simulink model "rpi_dc_motor_control"  (R2014a)
settings: Solver=FixedStepDiscrete  StartTime=0.0  StopTime=5000  FixedStep=0.001  RelTol=1e-3
undefined symbols (not defined in the file): DiscIntNeverNeededParam
settings Model: SimulationMode=external  ExtModeTrigDuration=200000  Creator=krecmich  LastModifiedBy=ses
settings OptimizationCC: ExpressionDepthLimit=2147483647  OptimizeModelRefInitCode=on  LifeSpan=1
settings DebuggingCC: UnderspecifiedInitializationDetection=Classic  StateNameClashWarn=warning
settings HardwareCC: ProdBitPerLong=64  ProdBitPerPointer=64  ProdIntDivRoundTo=Zero  ProdEndianess=LittleEndian  ProdWordSize=64  ProdHWDeviceType=Intel->x86-64
settings RTWCC: SystemTargetFile=ert_linux.tlc  MakeCommand="make_rtw OPT_OPTS=\"-O2 -ggdb -Wall\" CC=arm-linux-gnueabihf-gcc"  TemplateMakefile=ert_linux.tmf  Description=Linux Embedded Coder  GenerateReport=on  ProcessScript=ert_linux_make_rtw_hook  IncludeHyperlinkInReport=on  LaunchReport=on
settings RTWCC: CustomSource=|
  | rpi_gpclk.c
  | rpi_gpio.c
  | rpi_spi.c
settings CodeAppCC: IgnoreCustomStorageClasses=off  CustomSymbolStrType=$N$R$M  InternalIdentifier=Classic
settings STFCustomTargetCC: ModelReferenceCompliant=off  ConcurrentExecutionCompliant=off  GeneratePreprocessorConditionals=Use local settings  CombineOutputUpdateFcns=on  ERTCustomFileBanners=on  SupportContinuousTime=off  MATLABClassNameForMDSCustomization=Simulink.SoftwareTarget.ERTCustomization  GRTInterface=off  SystemTargetFile=ert_linux.tlc
settings ERTTargetCC: GenerateSampleERTMain=off  ModelReferenceCompliant=off  SupportNonInlinedSFcns=on  ERTCustomFileTemplate=ert_linux_file_process.tlc

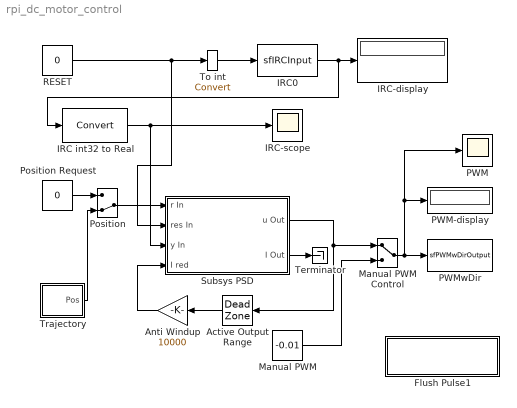
== system rpi_dc_motor_control ==
  "  RESET" : Constant  Value=0
      settings: OpenFcn=if get_param(gcbh,'value')=='0' set_param(gcbh,'value','1'); else set_param(gcbh,'value','0'); end;
  Active Output Range : DeadZone  LowerValue=-1  UpperValue=1  LinearizeAsGain=off
  Anti Windup : Gain  Gain=10000
  Flush Pulse1 : Subsystem  mask{target_ip_address='192.168.1.33'}
      mask prompts: target_ip_address "Target IP address"
      settings: OpenFcn=system(['./run_model.sh ', get_param(bdroot(gcbh),'name'),' ', get_param(gcbh,'target_ip_address')]);
      mask Display: disp('Double Click\n to run model on RPi')
  IRC int32 to Real : DataTypeConversion
  IRC-display : Display
  IRC-scope : Scope
      settings: TimeRange=50  YMin=-2100  YMax=2100  MaxDataPoints=200000
  IRC0 : S-Function  FunctionName=sfIRCInput  Parameters=Ts,chn-1,mode-1,gating-2,resetctrl-2,digfilter,reset_at_startup  EnableBusSupport=off  mask{chn=IRC0, mode=IRC, 4 edge detection (0), gating=Disabled (1), resetctrl=Value set by block input, digfilter=off, reset_at_startup=on, Ts=0.001}
      mask prompts: chn "IRC Channel"; mode "Counter Mode"; gating "Count Gating"; resetctrl "Reset Control"; digfilter "Digital Filter"; reset_at_startup "Reset at Startup"; Ts "Sample time (-1 for automatic)"
      mask TypeOptions chn: IRC0 | IRC1 | IRC2 | IRC3
      mask TypeOptions mode: IRC, 4 edge detection (0) | Bidirectional, rising edge (1) | Bidirectional, falling edge (2) | Bidirectional, either edge (3)
      mask TypeOptions gating: Value set by block input | Enabled (0) | Disabled (1) | Enabled if I0 input is 0 (2) | Enabled if I0 input is 1 (3)
      mask TypeOptions resetctrl: Value set by block input | Reset disabled (0) | Reset permanet (1) | Reset if I0 is 0 (2) | Reset if I0 is 1 (3) | Reset by rising edge of I0 (4) | Reset by falling edge of I0 (5) | Reset by either edge of I0 (6)
  Manual PWM : Constant  Value=-0.01
  Manual PWM Control : ManualSwitch
  PWM : Scope
      settings: TimeRange=50  YMin=-0.1  YMax=0.1  MaxDataPoints=200000
  PWM-display : Display
  PWMwDir : S-Function  FunctionName=sfPWMwDirOutput  Parameters=chn-1,pwm_freq,dir_do_bit-1  EnableBusSupport=off  mask{chn=PWM0, pwm_freq=20000, dir_do_bit=DO2}
      mask prompts: chn "PWM Output"; pwm_freq "PWM frequency (-1 from input)"; dir_do_bit "Direction DO Bit"
      mask TypeOptions chn: PWM0 | PWM1 | PWM2 | PWM3
      mask TypeOptions dir_do_bit: DO0 | DO1 | DO2 | DO3 | DO4 | DO5 | DO6 | DO7
  Position : ManualSwitch  CurrentSetting=0
  Position Request : Constant  Value=0
  Subsys PSD : Subsystem  mask(optimized PSD controller){P=0.0001, I=0.004, D=0.008, Ts=0.001}
      mask prompts: P "P proportional (P):"; I "I integral (I):"; D "D derivative (D):"; Ts "Sampling period (Ts):"
      mask help:
      | Type: Subsystem block.
      |
      | Description:
      |   Subsystem covers optimized PSD controller (PSD represents discretized PID).
      |
      | Requirements:
      |   Sampling period Ts.
      mask Help:
      | <b>Type:</b> Subsystem block.
      | <br><br>
      | <b>Description:</b><br>
      |   Subsystem covers optimized PSD controller (PSD represents discretized PID).
      | <br><br>
      | <b>Requirements:</b><br>
      |   Sampling period Ts.
      mask Display:
      | color('orange');disp('\n          Opt. PSD\n          Controller');
      | color('green');port_label('input', 1, 'w');
      | color('red');port_label('input', 2, ' RSTs');
      | color('lightblue');port_label('input', 3, 'r');
      | color('orange');port_label('input', 4, 'red I');
      | color('orange');port_label('output', 1, 'u ');
      | color('orange');port_label('output', 2, 'I  ');
      | color('red');disp('\n\n\n\n\n\n\n       P');
  Terminator : Terminator
  To int : DataTypeConversion
  Trajectory : Subsystem
  wires:
  IRC0/1 -> IRC int32 to Real/1, IRC-display/1
  IRC int32 to Real/1 -> Subsys PSD/3(y In), IRC-scope/1
  Manual PWM/1 -> Manual PWM Control/2
  Manual PWM Control/1 -> PWM/1, PWM-display/1, PWMwDir/1
  Subsys PSD/1(u Out) -> Active Output Range/1, Manual PWM Control/1
  "  RESET"/1 -> Subsys PSD/2(res In), To int/1
  Active Output Range/1 -> Anti Windup/1
  Anti Windup/1 -> Subsys PSD/4(I red)
  Position/1 -> Subsys PSD/1(r In)
  Position Request/1 -> Position/1
  To int/1 -> IRC0/1
  Trajectory/1(Pos) -> Position/2
  Subsys PSD/2(I Out) -> Terminator/1

== system rpi_dc_motor_control/Flush Pulse1 ==

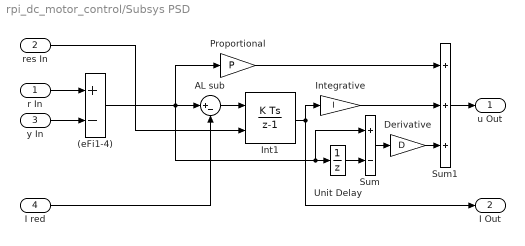
== system rpi_dc_motor_control/Subsys PSD ==
  r In : Inport  SampleTime=Ts
  res In : Inport  Port=2
  y In : Inport  Port=3  SampleTime=Ts
  I red : Inport  Port=4
  "  Derivative" : Gain  Gain=D  SaturateOnIntegerOverflow=on  OutDataTypeStr=Inherit: Same as input  ParamDataTypeStr=Inherit: Same as input
  (eFi1-4) : Sum  Inputs=+-  SaturateOnIntegerOverflow=on  InputSameDT=on  OutDataTypeStr=Inherit: Same as first input
  AL sub : Sum  Inputs=|+-  SaturateOnIntegerOverflow=on  InputSameDT=on  OutDataTypeStr=Inherit: Same as first input
  Int1 : DiscreteIntegrator  ExternalReset=level  SampleTime=-1  ICPrevOutput=DiscIntNeverNeededParam  ICPrevScaledInput=DiscIntNeverNeededParam
  Integrative : Gain  Gain=I  SaturateOnIntegerOverflow=on  OutDataTypeStr=Inherit: Same as input  ParamDataTypeStr=Inherit: Same as input
  Proportional : Gain  Gain=P  SaturateOnIntegerOverflow=on  OutDataTypeStr=Inherit: Same as input  ParamDataTypeStr=Inherit: Same as input
  Sum : Sum  Inputs=+-  SaturateOnIntegerOverflow=on  InputSameDT=on  OutDataTypeStr=Inherit: Same as first input
  Sum1 : Sum  Inputs=+++  SaturateOnIntegerOverflow=on  InputSameDT=on  OutDataTypeStr=Inherit: Same as first input
  Unit Delay : UnitDelay  SampleTime=Ts
  u Out : Outport
  I Out : Outport  Port=2
  wires:
  r In/1 -> (eFi1-4)/1
  y In/1 -> (eFi1-4)/2
  (eFi1-4)/1 -> Proportional/1, AL sub/1, Sum/1, Unit Delay/1
  "  Derivative"/1 -> Sum1/3
  Int1/1 -> I Out/1, Integrative/1
  Proportional/1 -> Sum1/1
  Sum1/1 -> u Out/1
  Sum/1 -> "  Derivative"/1
  Unit Delay/1 -> Sum/2
  res In/1 -> Int1/2
  AL sub/1 -> Int1/1
  I red/1 -> AL sub/2
  Integrative/1 -> Sum1/2

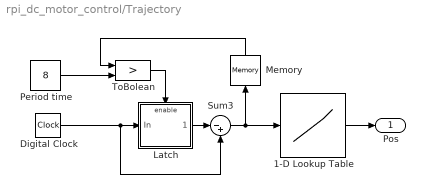
== system rpi_dc_motor_control/Trajectory ==
  1-D Lookup Table : Lookup_n-D  NumberOfTableDimensions=1  BreakpointsForDimension1="[0 3      5     6     6.1 8]"  Table="[0 2000 500 500 0    0]"  RndMeth=Simplest  InputSameDT=on
  Digital Clock : DigitalClock  SampleTime=0.001
  Latch : Subsystem  TreatAsAtomicUnit=on  mask(Latch){}
      mask help: Latch input signal.
      mask Display: disp('Latch')
  Memory : Memory
  Period time : Constant  Value=8
  Sum3 : Sum  Inputs=|-+  SaturateOnIntegerOverflow=on  InputSameDT=on  OutDataTypeStr=Inherit: Same as first input
  ToBolean : RelationalOperator  Operator=>
  Pos : Outport
  wires:
  Digital Clock/1 -> Sum3/2, Latch/1(In)
  Sum3/1 -> 1-D Lookup Table/1, Memory/1
  1-D Lookup Table/1 -> Pos/1
  Latch/1(" ") -> Sum3/1
  ToBolean/1 -> Latch/Enable
  Period time/1 -> ToBolean/2
  Memory/1 -> ToBolean/1

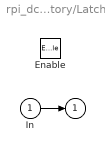
== system rpi_dc_motor_control/Trajectory/Latch ==
  In : Inport
  Enable : EnablePort
  " " : Outport  InitialOutput=0
  wires:
  In/1 -> " "/1
